simulink model "test15"  (R2021a)
settings: Solver=VariableStepAuto  StartTime=0.0  StopTime=tspan(end)  MaxStep=20/60/24  RelTol=1e-3
values from neighbouring files (symbols this model uses):
  cv_params = cv_p    [test15_script.m]
libraries: HORTISIM x4
settings Model: Creator=djoroya  LastModifiedBy=djoroya
settings DebuggingCC: UnconnectedInputMsg=none  UnconnectedOutputMsg=none  UnconnectedLineMsg=none

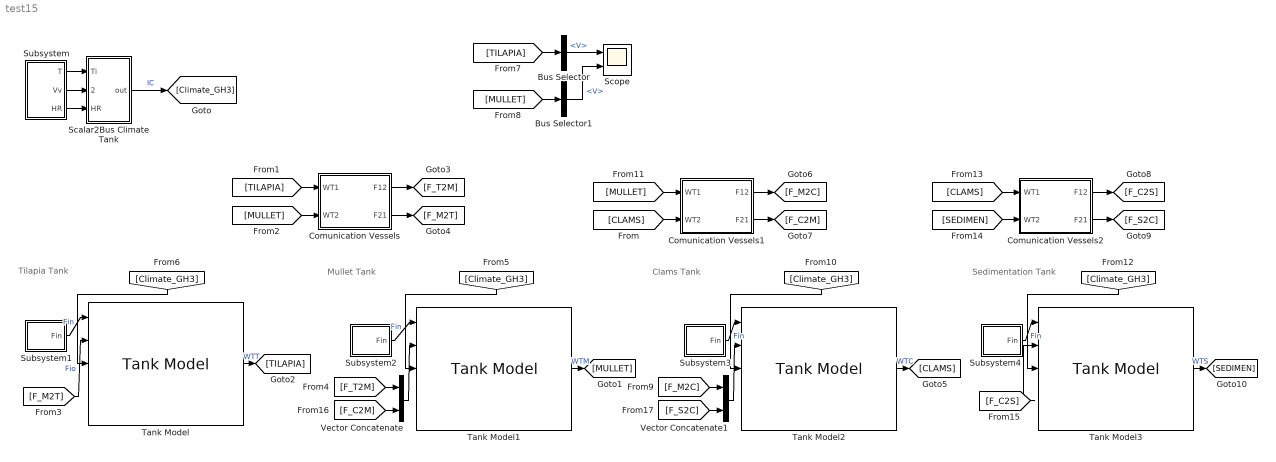
== system test15 ==
  note: Mullet Tank
  note: Tilapia Tank
  note: Clams Tank
  note: Sedimentation Tank
  Bus Selector : BusSelector  OutputSignals=V
  Bus Selector1 : BusSelector  OutputSignals=V
  Comunication Vessels : Subsystem  mask{params=cv_params}
  Comunication Vessels1 : Subsystem  mask{params=cv_params}
  Comunication Vessels2 : Subsystem  mask{params=cv_params}
  "Scalar2Bus Climate Tank " : Subsystem
  Scope : Scope  NumInputPorts=2
  Subsystem : Subsystem
  Subsystem1 : Subsystem
  Subsystem2 : Subsystem
  Subsystem3 : Subsystem
  Subsystem4 : Subsystem
  Tank Model : HORTISIM/Aquaculture/Models/Tank Model  x0=x0_tank_tilapia  params=tp_tilapia
      settings: SourceProductName=Horti Simulator
  Tank Model1 : HORTISIM/Aquaculture/Models/Tank Model  x0=x0_tank_mullet  params=tp_mullet
      settings: SourceProductName=Horti Simulator
      mask Display: image('water_tank.png'); % Use "Edit Image" on toolstrip to change.
  Tank Model2 : HORTISIM/Aquaculture/Models/Tank Model  x0=x0_tank_clams  params=tp_clams
      settings: SourceProductName=Horti Simulator
      mask Display: image('water_tank.png'); % Use "Edit Image" on toolstrip to change.
  Tank Model3 : HORTISIM/Aquaculture/Models/Tank Model  x0=x0_tank_sedim  params=tp_sedim
      settings: SourceProductName=Horti Simulator
      mask Display: image('water_tank.png'); % Use "Edit Image" on toolstrip to change.
  Vector Concatenate : Concatenate
  Vector Concatenate1 : Concatenate
  wires:
  Subsystem/3(HR) -> "Scalar2Bus Climate Tank "/3(HR)
  Subsystem/1(T) -> "Scalar2Bus Climate Tank "/1(Ti)
  Subsystem/2(Vv) -> "Scalar2Bus Climate Tank "/2(Speed)
  Subsystem1/1(Fin) -> Tank Model/1  "Fin"
  [F_M2T] -> Tank Model/2  "Fio"
  "Scalar2Bus Climate Tank "/1(out) -> [Climate_GH3]  "IC"
  [Climate_GH3] -> Tank Model/3
  Tank Model1/1 -> [MULLET]  "WTM"
  Tank Model/1 -> [TILAPIA]  "WTT"
  [TILAPIA] -> Comunication Vessels/1(WT1)
  [MULLET] -> Comunication Vessels/2(WT2)
  Comunication Vessels/1(F12) -> [F_T2M]
  Comunication Vessels/2(F21) -> [F_M2T]
  [Climate_GH3] -> Tank Model1/3
  Subsystem2/1(Fin) -> Tank Model1/1  "Fin"
  [TILAPIA] -> Bus Selector/1
  [MULLET] -> Bus Selector1/1
  Bus Selector/1 -> Scope/1  "<V>"
  Bus Selector1/1 -> Scope/2  "<V>"
  Comunication Vessels1/2(F21) -> [F_C2M]
  [CLAMS] -> Comunication Vessels1/2(WT2)
  Comunication Vessels1/1(F12) -> [F_M2C]
  [MULLET] -> Comunication Vessels1/1(WT1)
  [CLAMS] -> Comunication Vessels2/1(WT1)
  [SEDIMEN] -> Comunication Vessels2/2(WT2)
  Comunication Vessels2/1(F12) -> [F_C2S]
  Comunication Vessels2/2(F21) -> [F_S2C]
  Tank Model2/1 -> [CLAMS]  "WTC"
  Subsystem3/1(Fin) -> Tank Model2/1  "Fin"
  [Climate_GH3] -> Tank Model2/3
  Tank Model3/1 -> [SEDIMEN]  "WTS"
  Subsystem4/1(Fin) -> Tank Model3/1  "Fin"
  [Climate_GH3] -> Tank Model3/3
  [F_C2S] -> Tank Model3/2
  Vector Concatenate/1 -> Tank Model1/2
  [F_T2M] -> Vector Concatenate/1
  [F_C2M] -> Vector Concatenate/2
  Vector Concatenate1/1 -> Tank Model2/2
  [F_M2C] -> Vector Concatenate1/1
  [F_S2C] -> Vector Concatenate1/2

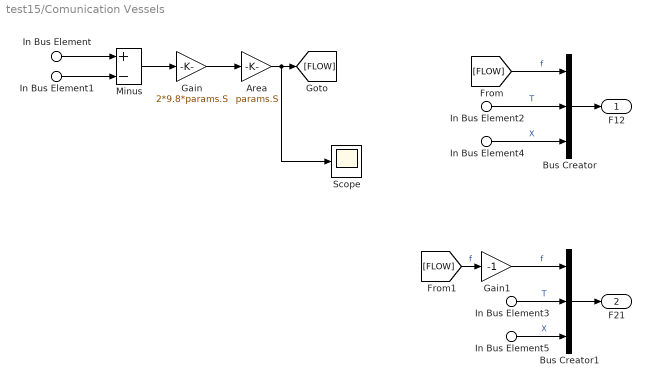
== system test15/Comunication Vessels ==
  In Bus Element : Inport  PortName=WT1  Element=h
  In Bus Element2 : Inport  PortName=WT1  Element=Fout.T
  In Bus Element4 : Inport  PortName=WT1  Element=Fout.X
  In Bus Element1 : Inport  Port=2  PortName=WT2  Element=h
  In Bus Element3 : Inport  Port=2  PortName=WT2  Element=Fout.T
  In Bus Element5 : Inport  Port=2  PortName=WT2  Element=Fout.X
  Area : Gain  Gain=params.S
  Bus Creator : BusCreator  Inputs=3  OutDataTypeStr=Bus: FLOW  NonVirtualBus=on
  Bus Creator1 : BusCreator  Inputs=3  OutDataTypeStr=Bus: FLOW  NonVirtualBus=on
  Gain : Gain  Gain=2*9.8*params.S
  Gain1 : Gain  Gain=-1
  Minus : Sum  Inputs=+-
  Scope : Scope
  F12 : Outport
  F21 : Outport  Port=2
  wires:
  In Bus Element/1 -> Minus/1
  In Bus Element1/1 -> Minus/2
  Minus/1 -> Gain/1
  Gain/1 -> Area/1
  Area/1 -> Scope/1, [FLOW]
  Bus Creator/1 -> F12/1
  [FLOW] -> Bus Creator/1  "f"
  In Bus Element2/1 -> Bus Creator/2  "T"
  In Bus Element4/1 -> Bus Creator/3  "X"
  Bus Creator1/1 -> F21/1
  Gain1/1 -> Bus Creator1/1  "f"
  In Bus Element3/1 -> Bus Creator1/2  "T"
  In Bus Element5/1 -> Bus Creator1/3  "X"
  [FLOW] -> Gain1/1  "f"

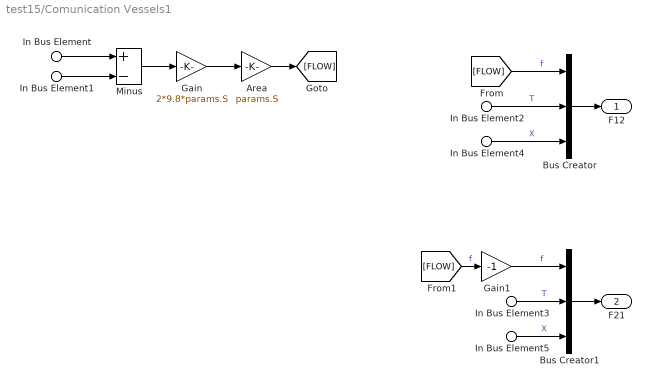
== system test15/Comunication Vessels1 ==
  In Bus Element : Inport  PortName=WT1  Element=h
  In Bus Element2 : Inport  PortName=WT1  Element=Fout.T
  In Bus Element4 : Inport  PortName=WT1  Element=Fout.X
  In Bus Element1 : Inport  Port=2  PortName=WT2  Element=h
  In Bus Element3 : Inport  Port=2  PortName=WT2  Element=Fout.T
  In Bus Element5 : Inport  Port=2  PortName=WT2  Element=Fout.X
  Area : Gain  Gain=params.S
  Bus Creator : BusCreator  Inputs=3  OutDataTypeStr=Bus: FLOW  NonVirtualBus=on
  Bus Creator1 : BusCreator  Inputs=3  OutDataTypeStr=Bus: FLOW  NonVirtualBus=on
  Gain : Gain  Gain=2*9.8*params.S
  Gain1 : Gain  Gain=-1
  Minus : Sum  Inputs=+-
  F12 : Outport
  F21 : Outport  Port=2
  wires:
  In Bus Element/1 -> Minus/1
  In Bus Element1/1 -> Minus/2
  Minus/1 -> Gain/1
  Gain/1 -> Area/1
  Area/1 -> [FLOW]
  Bus Creator/1 -> F12/1
  [FLOW] -> Bus Creator/1  "f"
  In Bus Element2/1 -> Bus Creator/2  "T"
  In Bus Element4/1 -> Bus Creator/3  "X"
  Bus Creator1/1 -> F21/1
  Gain1/1 -> Bus Creator1/1  "f"
  In Bus Element3/1 -> Bus Creator1/2  "T"
  In Bus Element5/1 -> Bus Creator1/3  "X"
  [FLOW] -> Gain1/1  "f"

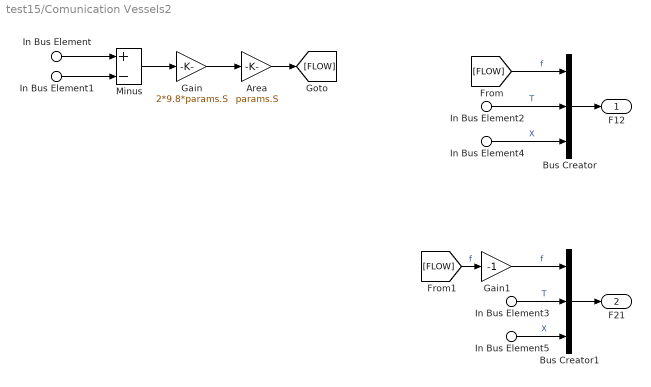
== system test15/Comunication Vessels2 ==
  In Bus Element : Inport  PortName=WT1  Element=h
  In Bus Element2 : Inport  PortName=WT1  Element=Fout.T
  In Bus Element4 : Inport  PortName=WT1  Element=Fout.X
  In Bus Element1 : Inport  Port=2  PortName=WT2  Element=h
  In Bus Element3 : Inport  Port=2  PortName=WT2  Element=Fout.T
  In Bus Element5 : Inport  Port=2  PortName=WT2  Element=Fout.X
  Area : Gain  Gain=params.S
  Bus Creator : BusCreator  Inputs=3  OutDataTypeStr=Bus: FLOW  NonVirtualBus=on
  Bus Creator1 : BusCreator  Inputs=3  OutDataTypeStr=Bus: FLOW  NonVirtualBus=on
  Gain : Gain  Gain=2*9.8*params.S
  Gain1 : Gain  Gain=-1
  Minus : Sum  Inputs=+-
  F12 : Outport
  F21 : Outport  Port=2
  wires:
  In Bus Element/1 -> Minus/1
  In Bus Element1/1 -> Minus/2
  Minus/1 -> Gain/1
  Gain/1 -> Area/1
  Area/1 -> [FLOW]
  Bus Creator/1 -> F12/1
  [FLOW] -> Bus Creator/1  "f"
  In Bus Element2/1 -> Bus Creator/2  "T"
  In Bus Element4/1 -> Bus Creator/3  "X"
  Bus Creator1/1 -> F21/1
  Gain1/1 -> Bus Creator1/1  "f"
  In Bus Element3/1 -> Bus Creator1/2  "T"
  In Bus Element5/1 -> Bus Creator1/3  "X"
  [FLOW] -> Gain1/1  "f"

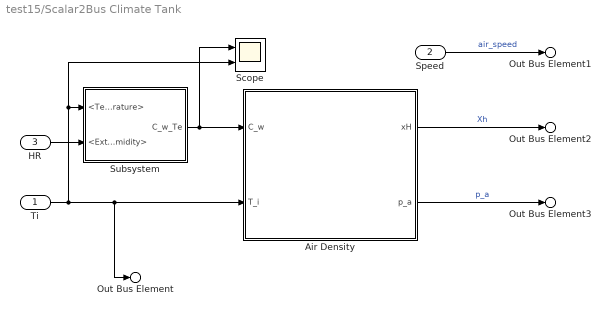
== system test15/Scalar2Bus Climate Tank  ==
  Ti : Inport
  Speed : Inport  Port=2
  HR : Inport  Port=3
  Air Density : MATLAB Function  TreatAsAtomicUnit=on
  Scope : Scope  NumInputPorts=2
  Subsystem : Subsystem
  Out Bus Element : Outport  PortName=out  Element=Temp.Tair
  Out Bus Element1 : Outport  PortName=out  Element=Gas.air_speed
  Out Bus Element2 : Outport  PortName=out  Element=Gas.Xh
  Out Bus Element3 : Outport  PortName=out  Element=Gas.p_a
  wires:
  Air Density/2(p_a) -> Out Bus Element3/1  "p_a"
  Air Density/1(xH) -> Out Bus Element2/1  "Xh"
  Speed/1 -> Out Bus Element1/1  "air_speed"
  Subsystem/1(C_w_Te) -> Scope/1, Air Density/1(C_w)
  Ti/1 -> Out Bus Element/1, Air Density/2(T_i), Scope/2, Subsystem/1(<Temperature>)
  HR/1 -> Subsystem/2(<Exterior Humidity>)

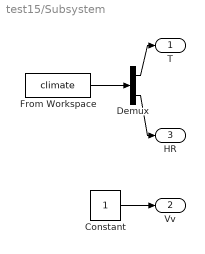
== system test15/Subsystem ==
  Constant : Constant
  Demux : Demux  Outputs=2
  From Workspace : FromWorkspace  VariableName=climate
  T : Outport
  Vv : Outport  Port=2
  HR : Outport  Port=3
  wires:
  Demux/1 -> T/1
  Demux/2 -> HR/1
  From Workspace/1 -> Demux/1
  Constant/1 -> Vv/1

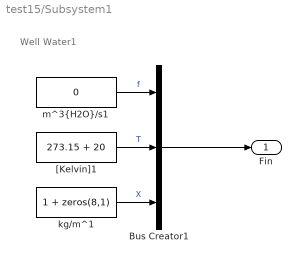
== system test15/Subsystem1 ==
  note: Well Water1
  Bus Creator1 : BusCreator  Inputs=3  OutDataTypeStr=Bus: FLOW  NonVirtualBus=on
  "[Kelvin]1" : Constant  Value=273.15 + 20
  kg/m^1 : Constant  Value=1 + zeros(8,1)
  "m^3{H2O}/s1" : Constant  Value=0
  Fin : Outport
  wires:
  Bus Creator1/1 -> Fin/1
  kg/m^1/1 -> Bus Creator1/3  "X"
  "[Kelvin]1"/1 -> Bus Creator1/2  "T"
  "m^3{H2O}/s1"/1 -> Bus Creator1/1  "f"

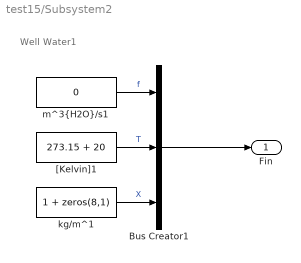
== system test15/Subsystem2 ==
  note: Well Water1
  Bus Creator1 : BusCreator  Inputs=3  OutDataTypeStr=Bus: FLOW  NonVirtualBus=on
  "[Kelvin]1" : Constant  Value=273.15 + 20
  kg/m^1 : Constant  Value=1 + zeros(8,1)
  "m^3{H2O}/s1" : Constant  Value=0
  Fin : Outport
  wires:
  Bus Creator1/1 -> Fin/1
  kg/m^1/1 -> Bus Creator1/3  "X"
  "[Kelvin]1"/1 -> Bus Creator1/2  "T"
  "m^3{H2O}/s1"/1 -> Bus Creator1/1  "f"

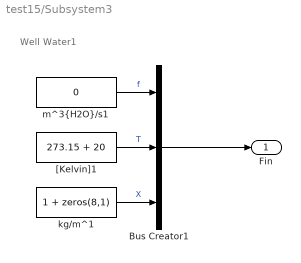
== system test15/Subsystem3 ==
  note: Well Water1
  Bus Creator1 : BusCreator  Inputs=3  OutDataTypeStr=Bus: FLOW  NonVirtualBus=on
  "[Kelvin]1" : Constant  Value=273.15 + 20
  kg/m^1 : Constant  Value=1 + zeros(8,1)
  "m^3{H2O}/s1" : Constant  Value=0
  Fin : Outport
  wires:
  Bus Creator1/1 -> Fin/1
  kg/m^1/1 -> Bus Creator1/3  "X"
  "[Kelvin]1"/1 -> Bus Creator1/2  "T"
  "m^3{H2O}/s1"/1 -> Bus Creator1/1  "f"

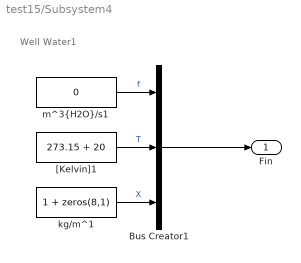
== system test15/Subsystem4 ==
  note: Well Water1
  Bus Creator1 : BusCreator  Inputs=3  OutDataTypeStr=Bus: FLOW  NonVirtualBus=on
  "[Kelvin]1" : Constant  Value=273.15 + 20
  kg/m^1 : Constant  Value=1 + zeros(8,1)
  "m^3{H2O}/s1" : Constant  Value=0
  Fin : Outport
  wires:
  Bus Creator1/1 -> Fin/1
  kg/m^1/1 -> Bus Creator1/3  "X"
  "[Kelvin]1"/1 -> Bus Creator1/2  "T"
  "m^3{H2O}/s1"/1 -> Bus Creator1/1  "f"

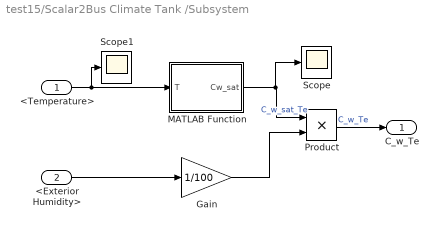
== system test15/Scalar2Bus Climate Tank /Subsystem ==
  <Temperature> : Inport
  <Exterior Humidity> : Inport  Port=2
  Gain : Gain  Gain=1/100
  MATLAB Function : MATLAB Function  TreatAsAtomicUnit=on
  Product : Product
  Scope : Scope
  Scope1 : Scope
  C_w_Te : Outport
  wires:
  Gain/1 -> Product/2
  MATLAB Function/1(Cw_sat) -> Scope/1, Product/1  "C_w_sat_Te"
  <Exterior Humidity>/1 -> Gain/1
  <Temperature>/1 -> MATLAB Function/1(T), Scope1/1
  Product/1 -> C_w_Te/1  "C_w_Te"

== matlab function test15/Scalar2Bus Climate Tank /Subsystem/MATLAB Function ==
  data: T input; Cw_sat output
function Cw_sat = fcn(T)

pws = exp(77.3450 + 0.0057*T - 7235 / T)/T^8.2;
Cw_sat = 0.0022*pws/T;

== matlab function test15/Scalar2Bus Climate Tank /Air Density ==
  data: C_w input; T_i input; xH output; p_a output
function [xH,p_a] =   Air(C_w,T_i)

% CONSTANTS
% =========  
atm = 101300; % standard atmospheric pressure [Pa]
R   = 8.3140; % gas constant [J/mol/K]
M_w = 0.0180; % molar mass of water [kg/mol]

%%
p_w = C_w*R.*T_i/M_w; % Partial pressure of water [Pa]
p_a = (atm - p_w);

xH = 0.62198* p_w /(p_a - p_w);
%%
